simulink model "test3"  (R2018b)
settings: Solver=ode45  StartTime=0.0  StopTime=0.01  RelTol=1e-3  EnableMultiTasking=on
libraries: commutil2 x2, commchan3 x1
settings Model: Creator=qiubo  LastModifiedBy=Aurora
settings DataIOCC: LimitDataPoints=on  SaveFormat=Array
settings OptimizationCC: LifeSpan=inf
settings DebuggingCC: UnderspecifiedInitializationDetection=Classic  MergeDetectMultiDrivingBlocksExec=none  SolverPrmCheckMsg=warning  StateNameClashWarn=warning  SFUnexpectedBacktrackingDiag=warning  SFNoUnconditionalDefaultTransitionDiag=warning  SFExecutionAtInitializationDiag=none
settings HardwareCC: ProdBitPerPointer=32  ProdBitPerSizeT=32  ProdBitPerPtrDiffT=32  ProdLargestAtomicFloat=None  ProdIntDivRoundTo=Undefined  ProdEndianess=Unspecified  ProdWordSize=32  ProdHWDeviceType=32-bit Generic
settings ModelReferenceCC: PropagateSignalLabelsOutOfModel=off
settings SFSimCC: SimUseLocalCustomCode=off
settings RTWCC: RTWUseLocalCustomCode=off
settings CodeAppCC: StateflowObjectComments=on
settings GRTTargetCC: TargetLangStandard=C89/C90 (ANSI)  GeneratePreprocessorConditionals=Disable all
settings ConfigComp: CovMetricSettings=dw  CovHtmlReporting=on  CovSaveCumulativeToWorkspaceVar=on  CovSaveSingleToWorkspaceVar=on  CovExternalEMLEnable=off

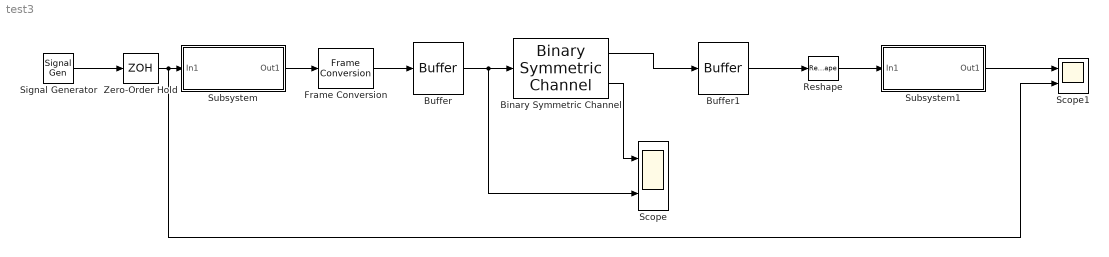
== system test3 ==
  Binary Symmetric Channel : commchan3/Binary Symmetric Channel  ErrorProbability=0.02  ErrorVectorOutputPort=on  OutputDataType=double  OutputDataTypeSL=double  Seed=71  SimulateUsing=Code generation
      settings: SourceProductName=Communications Toolbox  SourceProductBaseCode=CM
  Buffer : Buffer  N=1
  Buffer1 : Buffer  N=8
  Frame Conversion : FrameConversion
  Reshape : Reshape
  Scope : Scope  NumInputPorts=2
  Scope1 : Scope  NumInputPorts=2
  Signal Generator : SignalGenerator  Frequency=200
  Subsystem : Subsystem
  Subsystem1 : Subsystem
  Zero-Order Hold : ZeroOrderHold  SampleTime=1/8000
  wires:
  Signal Generator/1 -> Zero-Order Hold/1
  Subsystem/1(Out1) -> Frame Conversion/1
  Frame Conversion/1 -> Buffer/1
  Buffer/1 -> Scope/2, Binary Symmetric Channel/1
  Binary Symmetric Channel/1 -> Buffer1/1
  Binary Symmetric Channel/2 -> Scope/1
  Subsystem1/1(Out1) -> Scope1/1
  Buffer1/1 -> Reshape/1
  Reshape/1 -> Subsystem1/1(In1)
  Zero-Order Hold/1 -> Scope1/2, Subsystem/1(In1)

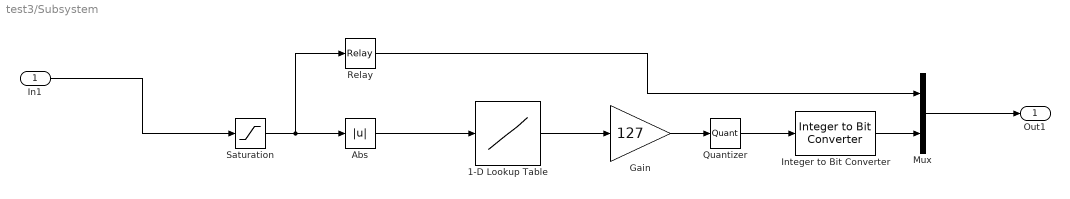
== system test3/Subsystem ==
  In1 : Inport
  1-D Lookup Table : Lookup_n-D  NumberOfTableDimensions=1  BreakpointsForDimension1=[0,1/128,1/64,1/32,1/16,1/8,1/4,1/2,1]  Table=[0:1/8:1]  RndMeth=Simplest  InputSameDT=on
  Abs : Abs
  Gain : Gain  Gain=127
  Integer to Bit Converter : commutil2/Integer to Bit Converter  nbits=7  signedInputValues=Unsigned  bitOrder=MSB first  outDtype=Same as input
      settings: SourceProductName=Communications Toolbox
  Mux : Mux  Inputs=2
  Quantizer : Quantizer  QuantizationInterval=1
  Relay : Relay
  Saturation : Saturate  UpperLimit=1  LowerLimit=-1
  Out1 : Outport
  wires:
  Quantizer/1 -> Integer to Bit Converter/1
  Gain/1 -> Quantizer/1
  In1/1 -> Saturation/1
  Saturation/1 -> Relay/1, Abs/1
  Abs/1 -> 1-D Lookup Table/1
  1-D Lookup Table/1 -> Gain/1
  Integer to Bit Converter/1 -> Mux/2
  Relay/1 -> Mux/1
  Mux/1 -> Out1/1

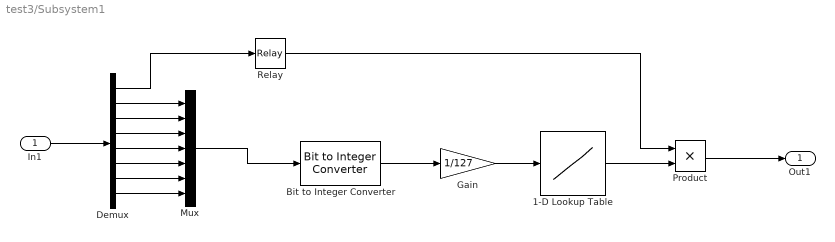
== system test3/Subsystem1 ==
  In1 : Inport
  1-D Lookup Table : Lookup_n-D  NumberOfTableDimensions=1  BreakpointsForDimension1=[0:1/8:1]  Table=[0,1/128,1/64,1/32,1/16,1/8,1/4,1/2,1]  RndMeth=Simplest  InputSameDT=on
  Bit to Integer Converter : commutil2/Bit to Integer Converter  nbits=7  bitOrder=MSB first  signedOutputValues=Unsigned  outDtype=Inherit via internal rule  outDtypeSigned=Inherit via internal rule
      settings: SourceProductName=Communications Toolbox
  Demux : Demux  Outputs=8
  Gain : Gain  Gain=1/127
  Mux : Mux  Inputs=7
  Product : Product
  Relay : Relay  OnSwitchValue=0.5  OffSwitchValue=0.5  OffOutputValue=-1
  Out1 : Outport
  wires:
  Demux/2 -> Mux/1
  Demux/3 -> Mux/2
  Demux/4 -> Mux/3
  Demux/5 -> Mux/4
  Demux/6 -> Mux/5
  Demux/7 -> Mux/6
  Demux/8 -> Mux/7
  Mux/1 -> Bit to Integer Converter/1
  Demux/1 -> Relay/1
  In1/1 -> Demux/1
  Bit to Integer Converter/1 -> Gain/1
  Gain/1 -> 1-D Lookup Table/1
  1-D Lookup Table/1 -> Product/2
  Product/1 -> Out1/1
  Relay/1 -> Product/1
